simulink model "u_expanded3"  (R2020b)
settings: Solver=VariableStepAuto  StartTime=0.0  StopTime=1  MaxStep=0.001  RelTol=1e-3
values from neighbouring files (symbols this model uses):
  c = 0    [init_params.m]
  m = M_eq    [LQR_params.m]    (also in init_params.m = 0.03)
  Ts = 0.01    [init_params.m]
undefined symbols (not defined in the file or in its folder): N, Th, xr_array
libraries: nesl_utility x8, fl_lib x5, sm_lib x3
settings Model: Creator=kaijunge  LastModifiedBy=kaijunge
settings SolverCC: AlgebraicLoopSolver=LineSearch

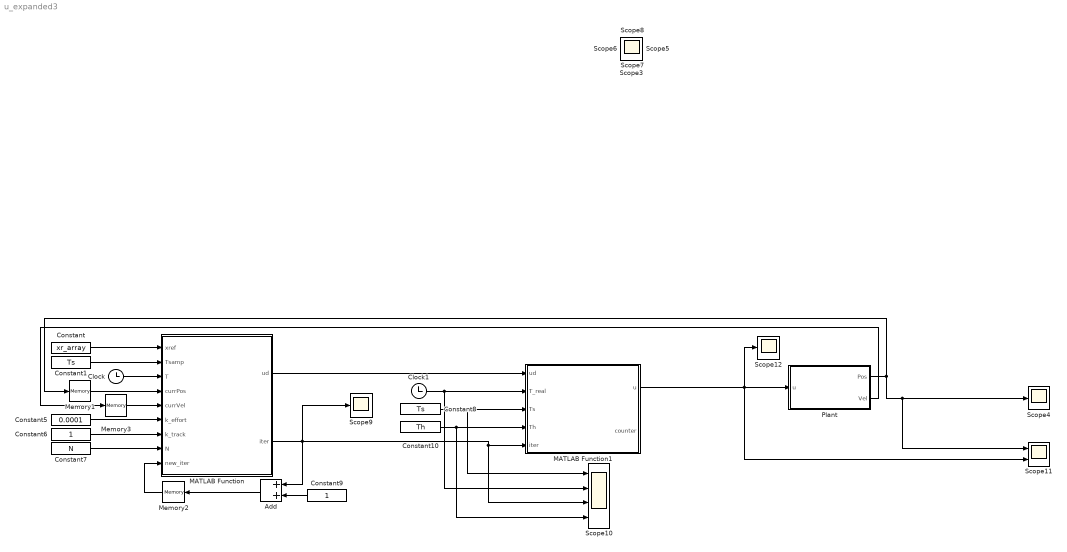
== system u_expanded3 ==
  Add : Sum
  Clock : Clock
  Clock1 : Clock
  Constant : Constant  Value=xr_array
  Constant1 : Constant  Value=Ts
  Constant10 : Constant  Value=Th
  Constant5 : Constant  Value=0.0001
  Constant6 : Constant
  Constant7 : Constant  Value=N
  Constant8 : Constant  Value=Ts
  Constant9 : Constant
  MATLAB Function : MATLAB Function  TreatAsAtomicUnit=on  SystemSampleTime=Th
  MATLAB Function1 : MATLAB Function  TreatAsAtomicUnit=on
  Memory1 : Memory
  Memory2 : Memory
  Memory3 : Memory
  Plant : Subsystem
  Scope10 : Scope  NumInputPorts=4
  Scope11 : Scope  NumInputPorts=2
  Scope{1..9,12} (10 alike) : Scope
  wires:
  Constant/1 -> MATLAB Function/1(xref)
  Constant1/1 -> MATLAB Function/2(Tsamp)
  Clock/1 -> MATLAB Function/3(T)
  Plant/1(Pos) -> Scope11/1, Scope4/1, Memory1/1
  Plant/2(Vel) -> Memory3/1
  Constant5/1 -> MATLAB Function/6(k_effort)
  Constant6/1 -> MATLAB Function/7(k_track)
  Constant7/1 -> MATLAB Function/8(N)
  Constant8/1 -> Scope10/1, MATLAB Function1/3(Ts)
  MATLAB Function/2(iter) -> Scope9/1, Scope10/3, MATLAB Function1/5(iter), Add/1
  Memory2/1 -> MATLAB Function/9(new_iter)
  Constant9/1 -> Add/2
  Add/1 -> Memory2/1
  Clock1/1 -> Scope10/2, MATLAB Function1/2(T_real)
  Constant10/1 -> Scope10/4, MATLAB Function1/4(Th)
  MATLAB Function/1(ud) -> MATLAB Function1/1(ud)
  MATLAB Function1/1(u) -> Scope12/1, Scope11/2, Plant/1(u)
  Memory1/1 -> MATLAB Function/4(currPos)
  Memory3/1 -> MATLAB Function/5(currVel)

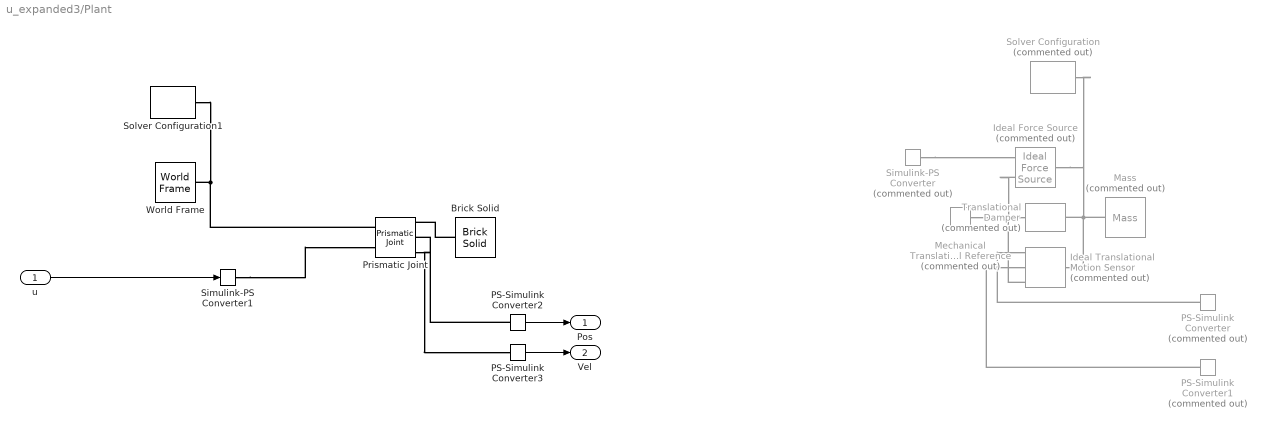
== system u_expanded3/Plant ==
  u : Inport
  Brick Solid : sm_lib/Body Elements/Brick Solid  GraphicAmbientColor=[0.15 0.15 0.15 1.0]  BasedOnType=Mass  BrickDimensions=[1 1 1]  BrickDimensionUnits=m  CenterOfMass=[0 0 0]  CenterOfMassUnits=m  GraphicDiffuseColor=[0.5 0.5 0.5]  Density=1000  DensityUnits=kg/m^3  DoExposeReferenceFrame=on  GraphicEmissiveColor=[0.0 0.0 0.0 1.0]  ExportEntireGeometry=off  SerializedFrames=<Frames/>  MarkerShape=Sphere  MarkerSize=10  GraphicType=FromGeometry  InertiaType=CalculateFromGeometry  Mass=1  MassUnits=kg  MomentsOfInertia=[1 1 1]  MomentsOfInertiaUnits=kg*m^2  GraphicOpacity=1.0  ProductsOfInertia=[0 0 0]  ProductsOfInertiaUnits=kg*m^2  GraphicShininess=75  GraphicSpecularColor=[0.5 0.5 0.5 1.0]  GraphicVisPropType=SimpleVisualProperties
  Ideal Force Source : fl_lib/Mechanical/Mechanical Sources/Ideal Force Source  Commented=on
  Ideal Translational Motion Sensor : fl_lib/Mechanical/Mechanical Sensors/Ideal Translational Motion Sensor  Commented=on  offset=0 m
  Mass : fl_lib/Mechanical/Translational Elements/Mass  Commented=on  mass=m kg  num_ports=foundation.enum.numPorts2.one  v_specify=off  v_priority=High  v=0 m/s  v_nominal_specify=off  v_nominal_unit=m/s  v_nominal_value=1  f_specify=off  f_priority=None  f=0 N  f_nominal_specify=off  f_nominal_unit=N  f_nominal_value=1
  Mechanical Translational Reference : fl_lib/Mechanical/Translational Elements/Mechanical Translational Reference  Commented=on
  PS-Simulink Converter : nesl_utility/PS-Simulink Converter  Commented=on  PhysicalDomain=network_engine_domain  SubClassName=ps_output  LeftPortType=input  RightPortType=output  PseudoPeriodic=off  Frequencies=[]  Unit=inherit  AffineConversion=off
  PS-Simulink Converter1 : nesl_utility/PS-Simulink Converter  Commented=on  PhysicalDomain=network_engine_domain  SubClassName=ps_output  LeftPortType=input  RightPortType=output  PseudoPeriodic=off  Frequencies=[]  Unit=inherit  AffineConversion=off
  PS-Simulink Converter2 : nesl_utility/PS-Simulink Converter  PhysicalDomain=network_engine_domain  SubClassName=ps_output  LeftPortType=input  RightPortType=output  PseudoPeriodic=off  Frequencies=[]  Unit=inherit  AffineConversion=off
  PS-Simulink Converter3 : nesl_utility/PS-Simulink Converter  PhysicalDomain=network_engine_domain  SubClassName=ps_output  LeftPortType=input  RightPortType=output  PseudoPeriodic=off  Frequencies=[]  Unit=inherit  AffineConversion=off
  Prismatic Joint : sm_lib/Joints/Prismatic Joint  JointMode=Normal  SenseConstraintForce=off  SenseConstraintForceX=off  SenseConstraintForceY=off  SenseConstraintForceZ=off  SenseConstraintTorque=off  SenseConstraintTorqueX=off  SenseConstraintTorqueY=off  SenseConstraintTorqueZ=off  SenseTotalForce=off  SenseTotalForceX=off  SenseTotalForceY=off  SenseTotalForceZ=off  SenseTotalTorque=off  SenseTotalTorqueX=off  SenseTotalTorqueY=off  SenseTotalTorqueZ=off  CompositeWrenchDir=FollowerOnBase  CompositeWrenchFrame=BaseFrame  EquilibriumPosition=0  EquilibriumPositionUnits=m  SpringStiffness=0  SpringStiffnessUnits=N/m  DampingCoefficient=0  DampingCoefficientUnits=N/(m/s)  TorqueActuationMode=InputTorque  MotionActuationMode=ComputedMotion  SensePosition=on  SenseVelocity=on  SenseAcceleration=off  SenseTorqueForce=off  SenseLowerLimitTorqueForce=off  SenseUpperLimitTorqueForce=off  LowerLimitSpecify=off  LowerLimitBound=-1  LowerLimitBoundUnits=m  LowerLimitStiffness=1e6  LowerLimitStiffnessUnits=N/m  LowerLimitDamping=1e3  LowerLimitDampingUnits=N/(m/s)  LowerLimitTransitionRegionWidth=1e-4  LowerLimitTransitionRegionWidthUnits=m  UpperLimitSpecify=off  UpperLimitBound=1  UpperLimitBoundUnits=m  UpperLimitStiffness=1e6  UpperLimitStiffnessUnits=N/m  UpperLimitDamping=1e3  UpperLimitDampingUnits=N/(m/s)  UpperLimitTransitionRegionWidth=1e-4  UpperLimitTransitionRegionWidthUnits=m  PositionTargetSpecify=off  PositionTargetPriority=High  PositionTargetValue=0  PositionTargetValueUnits=m  VelocityTargetSpecify=off  VelocityTargetPriority=High  VelocityTargetValue=0  VelocityTargetValueUnits=m/s
  Simulink-PS Converter : nesl_utility/Simulink-PS Converter  Commented=on  PhysicalDomain=network_engine_domain  SubClassName=ps_input  LeftPortType=input  RightPortType=output  PseudoPeriodic=off  Frequencies=[]  NoiseDistribution=none  NoiseParameters=[]  Unit=1  AffineConversion=off  FilteringAndDerivatives=provide  SimscapeFilterOrder=1  InputFilterTimeConstant=0.001  UdotUserProvided=0
  Simulink-PS Converter1 : nesl_utility/Simulink-PS Converter  PhysicalDomain=network_engine_domain  SubClassName=ps_input  LeftPortType=input  RightPortType=output  PseudoPeriodic=off  Frequencies=[]  NoiseDistribution=none  NoiseParameters=[]  Unit=1  AffineConversion=off  FilteringAndDerivatives=provide  SimscapeFilterOrder=1  InputFilterTimeConstant=0.001  UdotUserProvided=0
  Solver Configuration : nesl_utility/Solver Configuration  Commented=on  PhysicalDomain=network_engine_domain  SubClassName=solver  LeftPortType=input  RightPortType=generic  Tones=[]  Harmonics=[]  SimulateNoise=off  Profile=off  UseLocalSampling=off  EnableSwitchedLinearOptims=on  FrequencyDomain=off  UseCCode=off  RelTol=0.001  AbsTol=1e-06  MinStep=1e-09  ToWorkspace=off  RevertToSquareIcSolve=off  NumHomotopyIterations=100  PhasorMode=off  PhasorModeNumHarmonics=1  DoDC=off  ResidualTolerance=1e-09  UseLocalSolver=off  LocalSolverChoice=NE_BACKWARD_EULER_ADVANCER  LocalSolverSampleTime=0.001  DoFixedCost=off  MaxNonlinIter=3  MaxModeIter=2  ComputeImpulses=off  ImpulseIterations=2  LinearAlgebra=auto  EquationFormulation=NE_TIME_EF  DelaysMemoryBudget=1024  AutomaticFiltering=on  FilteringTimeConstant=0.001  PartitionStorageMethod=AS_NEEDED  PartitionMemoryBudget=1024  PartitionMethod=ROBUST
  Solver Configuration1 : nesl_utility/Solver Configuration  PhysicalDomain=network_engine_domain  SubClassName=solver  LeftPortType=input  RightPortType=generic  Tones=[]  Harmonics=[]  SimulateNoise=off  Profile=off  UseLocalSampling=off  EnableSwitchedLinearOptims=on  FrequencyDomain=off  UseCCode=off  RelTol=0.001  AbsTol=1e-06  MinStep=1e-09  ToWorkspace=off  RevertToSquareIcSolve=off  NumHomotopyIterations=100  PhasorMode=off  PhasorModeNumHarmonics=1  DoDC=off  ResidualTolerance=1e-09  UseLocalSolver=off  LocalSolverChoice=NE_BACKWARD_EULER_ADVANCER  LocalSolverSampleTime=0.001  DoFixedCost=off  MaxNonlinIter=3  MaxModeIter=2  ComputeImpulses=off  ImpulseIterations=2  LinearAlgebra=auto  EquationFormulation=NE_TIME_EF  DelaysMemoryBudget=1024  AutomaticFiltering=on  FilteringTimeConstant=0.001  PartitionStorageMethod=AS_NEEDED  PartitionMemoryBudget=1024  PartitionMethod=ROBUST
  Translational Damper : fl_lib/Mechanical/Translational Elements/Translational Damper  Commented=on  D=c N/(m/s)  v_specify=off  v_priority=None  v=0 m/s  v_nominal_specify=off  v_nominal_unit=m/s  v_nominal_value=1  f_specify=off  f_priority=None  f=0 N  f_nominal_specify=off  f_nominal_unit=N  f_nominal_value=1
  World Frame : sm_lib/Frames and Transforms/World Frame
  Pos : Outport
  Vel : Outport  Port=2
  wires:
  PS-Simulink Converter2/1 -> Pos/1
  u/1 -> Simulink-PS Converter1/1
  PS-Simulink Converter3/1 -> Vel/1
  connections:
  PS-Simulink Converter/LConn1 -- Ideal Translational Motion Sensor/RConn3
  PS-Simulink Converter1/LConn1 -- Ideal Translational Motion Sensor/RConn2
  Simulink-PS Converter/RConn1 -- Ideal Force Source/RConn1
  Mass/LConn1 -- Solver Configuration/RConn1 -- Ideal Force Source/LConn1 -- Ideal Translational Motion Sensor/LConn1 -- Translational Damper/RConn1
  Mechanical Translational Reference/LConn1 -- Ideal Force Source/RConn2 -- Ideal Translational Motion Sensor/RConn1 -- Translational Damper/LConn1
  World Frame/RConn1 -- Solver Configuration1/RConn1 -- Prismatic Joint/LConn1
  Brick Solid/RConn1 -- Prismatic Joint/RConn1
  Simulink-PS Converter1/RConn1 -- Prismatic Joint/LConn2
  PS-Simulink Converter2/LConn1 -- Prismatic Joint/RConn2
  Prismatic Joint/RConn3 -- PS-Simulink Converter3/LConn1

== matlab function u_expanded3/MATLAB Function ==
  data: xref input; ud output size=[1000, 1]; Tsamp input; T input; currPos input; currVel input; k_effort input; k_track input; N input; iter output; new_iter input
function [ud,iter]  = trajectory(xref, Tsamp, T, currPos, currVel, k_effort, k_track, N, new_iter)

% number of data points
N = double(N);

% reference x = step funciton 
currT_index = int32(T/Tsamp)+1;
xref = xref(currT_index:currT_index+N);

% initial condition
x0 = [currPos currVel];

A = [1 Tsamp; 0 1];
B = [0; Tsamp];

mat = zeros(2, N);

for i = 1:N
    mat(:,i) = (A^(i-1))*B;
end




H = 2*eye(2*N-1); % x2 to counteract the 1/2 coefficient in the solver

for i = 1:2*N-1 
    if i <= N
        H(i,i) = k_track*H(i,i);    
    else
        H(i,i) = k_effort*H(i,i);
    end
end

f = zeros(2*N-1,1);

for i = 1:N
    f(i) = -2*k_track*xref(i);
end

Aineq = [];
bineq = [];
Aeq = zeros(2*N-1);
beq = zeros(2*N-1, 1);
lb = zeros(2*N-1,1);
ub = zeros(2*N-1,1);

% set values in Aeq
Aeq(1,1) = 1;

for i = 2:N
    Aeq(i,i) = -1;
end

for i = 2:N
    Aeq(i, 1) = [1,0]*A^(i-1)*[1;0]; 
    
    p = zeros(1, N-1);
    p(1:i-1) = flip(mat(1, 1:i-1));
    Aeq(i,N+1:end) = p;
end

beq(1) = x0(1);
for i = 2:N
    beq(i) = -1*[1,0]*A^(i-1)*[0;1]*x0(2);
end

u_lim = Tsamp*1000;
for i = 1:2*N-1
    if i <= N
        lb(i) = -inf;
        ub(i) = inf;
    else
        lb(i) = -1*u_lim;
        ub(i) = u_lim;
    end
end

%x0 = zeros(2*N-1,1);
%options = optimoptions('quadprog','Algorithm','active-set');

coder.extrinsic('quadprog');
z = quadprog(H,f,Aineq,bineq,Aeq,beq,lb,ub);%,x0,options);

ud = zeros(1000, 1);
for i = 1:N-1
    ud(i) = z(N+i);
end
%ud = zeros(199, 1);

iter = new_iter;

== matlab function u_expanded3/MATLAB Function1 ==
  data: ud input size=[1000, 1]; u output; T_real input; counter output; Ts input; Th input; iter input
function [u, counter] = u_selector(ud, T_real, Ts, Th, iter)

counter = floor((T_real - Th*iter)/Ts)+1;
u = ud(counter);
